simulink library "csu_cpt_chamber_pressure_throttle_cmd_lib"  (R2014b)
settings: Solver=ode45  StartTime=0.0  StopTime=10.0  RelTol=1e-3
undefined symbols (not defined in the file or in its folder): egc_chamber_pressure_to_thrust, egc_pc_derivative_gain, egc_pc_integral_gain, egc_pc_proportional_gain
libraries: simulink x1, util_info_lib x1
settings Model: Creator=escrane  LastModifiedBy=mstewart

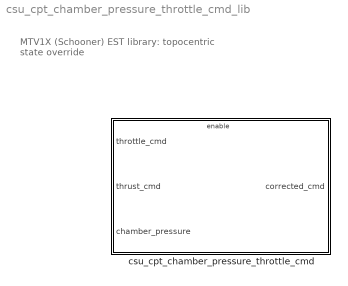
== system csu_cpt_chamber_pressure_throttle_cmd_lib ==
  note: MTV1X (Schooner) EST library:
      | topocentric state override
  csu_cpt_chamber_pressure_throttle_cmd : Subsystem

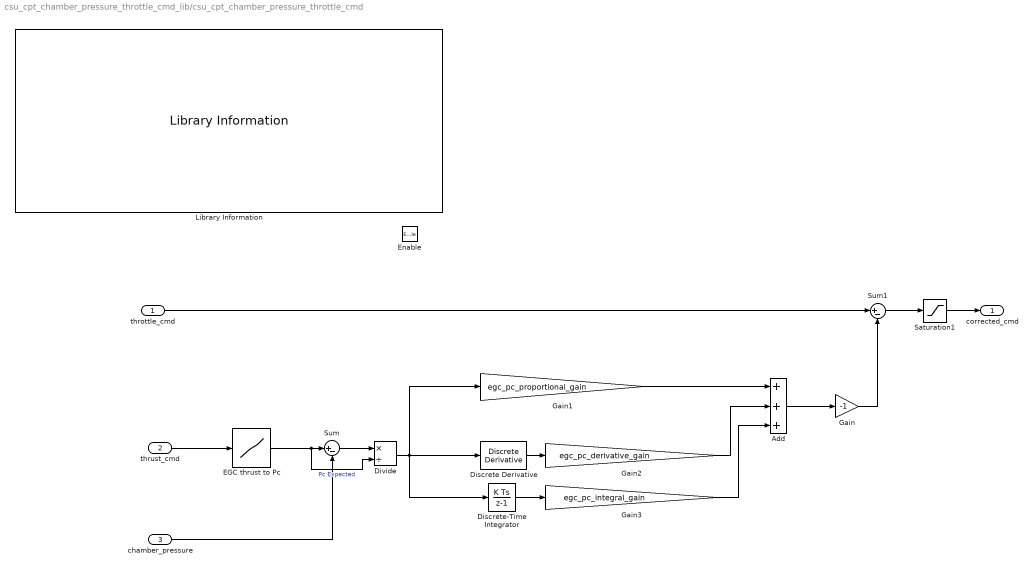
== system csu_cpt_chamber_pressure_throttle_cmd_lib/csu_cpt_chamber_pressure_throttle_cmd ==
  throttle_cmd : Inport
  thrust_cmd : Inport  Port=2
  chamber_pressure : Inport  Port=3
  Enable : EnablePort
  Add : Sum  Inputs=+++
  Discrete Derivative : simulink/Discrete/Discrete Derivative  gainval=1.0  ICPrevScaledInput=0.0  InputProcessing=Inherited  OutMin=[]  OutMax=[]  OutDataType=fixdt(1, 16)  OutScaling=2^-10  DoSatur=off
  Discrete-Time Integrator : DiscreteIntegrator  InitialConditionSetting=State (most efficient)  SampleTime=-1
  Divide : Product  Inputs=*/
  "EGC thrust to Pc " : Lookup  InputValues=egc_chamber_pressure_to_thrust(:,2)  Table=egc_chamber_pressure_to_thrust(:,1)  LookUpMeth=Interpolation-Use End Values
  Gain : Gain  Gain=-1
  Gain1 : Gain  Gain=egc_pc_proportional_gain
  Gain2 : Gain  Gain=egc_pc_derivative_gain
  Gain3 : Gain  Gain=egc_pc_integral_gain
  Library Information : util_info_lib/Library Information  owner='NONE'
  Saturation1 : Saturate  UpperLimit=1  LowerLimit=0
  Sum : Sum  Inputs=|+-
  Sum1 : Sum  Inputs=|+-
  "corrected_cmd " : Outport
  wires:
  Add/1 -> Gain/1
  Gain2/1 -> Add/2
  Gain1/1 -> Add/1
  Discrete Derivative/1 -> Gain2/1
  Sum1/1 -> Saturation1/1
  throttle_cmd/1 -> Sum1/1
  "EGC thrust to Pc "/1 -> Divide/2, Sum/1  "Pc Expected"
  thrust_cmd/1 -> "EGC thrust to Pc "/1
  Sum/1 -> Divide/1
  Divide/1 -> Discrete-Time Integrator/1, Gain1/1, Discrete Derivative/1
  chamber_pressure/1 -> Sum/2
  Gain/1 -> Sum1/2
  Saturation1/1 -> "corrected_cmd "/1
  Gain3/1 -> Add/3
  Discrete-Time Integrator/1 -> Gain3/1
